simulink model "Quaternions_Method_merge"  (R2021b)
settings: Solver=VariableStepAuto  StartTime=0.0  StopTime=Time  FixedStep=1e-1  RelTol=1e-13  AbsTol=1e-8
values from neighbouring files (symbols this model uses):
  a = 8.6251e+06    (= 8625100)    [Main.m]
  c = 299792*10^3    (= 299792000)    [Main.m]
  e = 0.1195    [Main.m]
  f_mag = 5    [Main.m]
  H_0 = sqrt((g_1_0)^2 + (g_1_1)^2 + (h_1_1)^2)    [Main.m]
  i = 0.3815    [Main.m]
  MB = [2000; 0.3; 1; 0.12].*1e-2    [Main.m]
  mr = 1.2 * 0.0001    (= 0.00012)    [Main.m]
  muP = G*Mt    (= 398527110340000)    [Main.m]
  omega_0 = [om_x, om_y, om_z]    [Main.m]
  p_acc = deg2rad(5)    [Main.m]
  RD = 0.1*ones(1,10)    [Main.m]
  RS_MB = 0.5    [Main.m]
  RS_SP = 0.1    [Main.m]
  SP = [2000; 0.3; 1; 0.12].*1e-2    [Main.m]
  theta0 = 0    [Main.m]
  w_E = (2*pi)/(24*3600)    (= 7.27220521664e-05)    [Main.m]
undefined symbols (not defined in the file or in its folder): A_BN_0, A_rw, A_rw_star, magnitude, sig_b, sig_n, T, t_sample
libraries: matrix_library x14, vrlib x8, simulink x2, simulink_extras x1
(part 4 of 4)

== system Quaternions_Method_merge/Enviroment/Solar Radiation Perturbation/Sum forces/determine highlighted area/creazione della matrice che ha per colonne i vettori distanza tra il CM del MB e i centri geom delle aree illuminate dal sole /creazione raggi vettore tra CM MB e centro facce illuminate della faccia che ha come normale l'asse j/If Action Subsystem3 ==
  Areas_vect : Inport
  MB : Inport  Port=2
  Action Port : ActionPort  ActionPortLabel=if(u1<0 & u2<0)
  Add : Sum  Inputs=+|-
  Add1 : Sum  Inputs=+|-
  Add2 : Sum
  Demux : Demux  Outputs=3
  Demux2 : Demux
  Divide : Product  Inputs=*/
  Divide1 : Product  Inputs=*/
  Gain{,1..3} (4 alike) : Gain  Gain=1/2
  Gain4 : Gain  Gain=-1
  Gain5 : Gain  Gain=-1
  Ground : Ground
  Ground1 : Ground
  Mux : Mux  Inputs=3
  Mux1 : Mux  Inputs=3
  Reshape : Reshape  OutputDimensionality=Column vector (2-D)
  Reshape2 : Reshape  OutputDimensionality=Column vector (2-D)
  Reshape3 : Reshape  OutputDimensionality=Column vector (2-D)
  Terminator{1..2,8..9} (4 alike) : Terminator
  r_cface_cluce_x_neg_z_neg : Outport
  wires:
  Add1/1 -> Gain4/1
  Gain4/1 -> Mux1/1
  Demux/3 -> Terminator8/1
  Demux/1 -> Terminator9/1
  Add2/1 -> r_cface_cluce_x_neg_z_neg/1
  Reshape3/1 -> Add2/2
  Reshape2/1 -> Add2/1
  [a_MB] -> Gain2/1
  Divide1/1 -> Gain3/1
  Gain2/1 -> Add1/1
  Gain3/1 -> Add1/2
  Ground/1 -> Mux1/3, Mux1/2
  Mux1/1 -> Reshape3/1  "raggio vettore che collega il centro geom della faccia con il centro geom della faccia illuminata dal sole lungo -i"
  [h_MB] -> Divide1/2
  Reshape/1 -> Demux/1
  Ground1/1 -> Mux/1, Mux/2
  Areas_vect/1 -> Reshape/1
  [a_MB] -> Divide/2
  Gain/1 -> Add/1
  [h_MB] -> Gain/1
  Demux/2 -> Divide/1, Divide1/1
  Gain1/1 -> Add/2
  Mux/1 -> Reshape2/1  "raggio vettore che collega il centro geom della faccia con il centro geom della faccia illuminata dal sole lungo -k"
  Divide/1 -> Gain1/1
  Add/1 -> Gain5/1
  Gain5/1 -> Mux/3
  Demux2/1 -> Terminator2/1
  Demux2/2 -> [a_MB]
  MB/1 -> Demux2/1
  Demux2/3 -> Terminator1/1
  Demux2/4 -> [h_MB]

== system Quaternions_Method_merge/Enviroment/Solar Radiation Perturbation/Sum forces/determine highlighted area/creazione della matrice che ha per colonne i vettori distanza tra il CM del MB e i centri geom delle aree illuminate dal sole /creazione raggi vettore tra CM MB e centro facce illuminate della faccia che ha come normale l'asse j/If Action Subsystem4 ==
  Action Port : ActionPort  ActionPortLabel=else
  Constant : Constant  Value=[0;0;0]
  Out1 : Outport
  wires:
  Constant/1 -> Out1/1

== system Quaternions_Method_merge/Enviroment/Solar Radiation Perturbation/Sum forces/determine highlighted area/creazione della matrice che ha per colonne i vettori distanza tra il CM del MB e i centri geom delle aree illuminate dal sole /creazione raggi vettore tra CM MB e centro facce illuminate della faccia che ha come normale l'asse j/If Action Subsystem5 ==
  Action Port : ActionPort  ActionPortLabel=else
  Constant : Constant  Value=[0;0;0]
  Out1 : Outport
  wires:
  Constant/1 -> Out1/1

== system Quaternions_Method_merge/Enviroment/Solar Radiation Perturbation/Sum forces/determine highlighted area/creazione della matrice che ha per colonne i vettori distanza tra il CM del MB e i centri geom delle aree illuminate dal sole /creazione raggi vettore tra CM MB e centro facce illuminate della faccia che ha come normale l'asse j/If Action Subsystem6 ==
  Action Port : ActionPort  ActionPortLabel=else
  Constant : Constant  Value=[0;0;0]
  Out1 : Outport
  wires:
  Constant/1 -> Out1/1

== system Quaternions_Method_merge/Enviroment/Solar Radiation Perturbation/Sum forces/determine highlighted area/creazione della matrice che ha per colonne i vettori distanza tra il CM del MB e i centri geom delle aree illuminate dal sole /creazione raggi vettore tra CM MB e centro facce illuminate della faccia che ha come normale l'asse j/If Action Subsystem7 ==
  Action Port : ActionPort  ActionPortLabel=else
  Constant : Constant  Value=[0;0;0]
  Out1 : Outport
  wires:
  Constant/1 -> Out1/1

== system Quaternions_Method_merge/Enviroment/Solar Radiation Perturbation/Sum forces/determine highlighted area/creazione della matrice che ha per colonne i vettori distanza tra il CM del MB e i centri geom delle aree illuminate dal sole /creazione raggi vettore tra CM MB e centro facce illuminate della faccia che ha come normale l'asse j/creating distance between cm MB and centro geom lato1 ==
  MB : Inport
  Demux : Demux
  Ground : Ground
  Mux : Mux  Inputs=3
  Reshape : Reshape  OutputDimensionality=Column vector (2-D)
  Terminator : Terminator
  Terminator1 : Terminator
  Terminator2 : Terminator
  Out1 : Outport
  wires:
  Reshape/1 -> Out1/1
  Mux/1 -> Reshape/1
  Demux/4 -> Mux/3
  MB/1 -> Demux/1
  Demux/1 -> Terminator/1
  Demux/2 -> Terminator1/1
  Demux/3 -> Terminator2/1
  Ground/1 -> Mux/1, Mux/2

== system Quaternions_Method_merge/Enviroment/Solar Radiation Perturbation/Sum forces/determine highlighted area/creazione della matrice che ha per colonne i vettori distanza tra il CM del MB e i centri geom delle aree illuminate dal sole /creazione raggi vettore tra CM MB e centro facce illuminate della faccia che ha come normale l'asse k/If Action Subsystem ==
  Areas_vect : Inport
  MB : Inport  Port=2
  Action Port : ActionPort  ActionPortLabel=if(u1>0 & u2>0)
  Add : Sum  Inputs=+|-
  Add1 : Sum  Inputs=+|-
  Add2 : Sum
  Demux : Demux  Outputs=3
  Demux1 : Demux  Outputs=3
  Demux2 : Demux
  Divide : Product  Inputs=*/
  Divide1 : Product  Inputs=*/
  Gain{,1..3} (4 alike) : Gain  Gain=1/2
  Ground : Ground
  Ground1 : Ground
  Mux : Mux  Inputs=3
  Mux1 : Mux  Inputs=3
  Reshape{,1..3} (4 alike) : Reshape  OutputDimensionality=Column vector (2-D)
  Terminator{,1..3,8..9} (6 alike) : Terminator
  r_cface_cluce_xy_pos : Outport
  wires:
  Add/1 -> Mux/2
  Divide/1 -> Gain1/1
  Mux/1 -> Reshape2/1  "raggio vettore che collega il centro geom della faccia con il centro geom della faccia illuminata dal sole lungo j"
  Gain1/1 -> Add/2
  Demux/3 -> Divide/1
  [b_MB] -> Gain/1
  Gain/1 -> Add/1
  [a_MB] -> Divide/2
  Areas_vect/1 -> Reshape/1, Reshape1/1
  Ground1/1 -> Mux/1, Mux/3
  Reshape/1 -> Demux/1
  Add1/1 -> Mux1/1
  [b_MB] -> Divide1/2
  Mux1/1 -> Reshape3/1  "raggio vettore che collega il centro geom della faccia con il centro geom della faccia illuminata dal sole lungo x"
  Ground/1 -> Mux1/2, Mux1/3
  Demux1/3 -> Divide1/1
  Gain3/1 -> Add1/2
  Gain2/1 -> Add1/1
  Reshape1/1 -> Demux1/1
  Divide1/1 -> Gain3/1
  [a_MB] -> Gain2/1
  Reshape2/1 -> Add2/1
  Reshape3/1 -> Add2/2
  Add2/1 -> r_cface_cluce_xy_pos/1
  Demux1/1 -> Terminator/1
  Demux1/2 -> Terminator1/1
  Demux/1 -> Terminator9/1
  Demux/2 -> Terminator8/1
  MB/1 -> Demux2/1
  Demux2/1 -> Terminator2/1
  Demux2/2 -> [a_MB]
  Demux2/3 -> [b_MB]
  Demux2/4 -> Terminator3/1

== system Quaternions_Method_merge/Enviroment/Solar Radiation Perturbation/Sum forces/determine highlighted area/creazione della matrice che ha per colonne i vettori distanza tra il CM del MB e i centri geom delle aree illuminate dal sole /creazione raggi vettore tra CM MB e centro facce illuminate della faccia che ha come normale l'asse k/If Action Subsystem1 ==
  Areas_vect : Inport
  MB : Inport  Port=2
  Action Port : ActionPort  ActionPortLabel=if(u1>0 & u2<0)
  Add : Sum  Inputs=+|-
  Add1 : Sum  Inputs=+|-
  Add2 : Sum
  Demux : Demux  Outputs=3
  Demux1 : Demux  Outputs=3
  Demux2 : Demux
  Divide : Product  Inputs=*/
  Divide1 : Product  Inputs=*/
  Gain{,1..3} (4 alike) : Gain  Gain=1/2
  Gain4 : Gain  Gain=-1
  Ground : Ground
  Ground1 : Ground
  Mux : Mux  Inputs=3
  Mux1 : Mux  Inputs=3
  Reshape{,1..3} (4 alike) : Reshape  OutputDimensionality=Column vector (2-D)
  Terminator{,1..3,8..9} (6 alike) : Terminator
  r_cface_cluce_xpos_y_neg : Outport
  wires:
  Add/1 -> Gain4/1
  Divide/1 -> Gain1/1
  Mux/1 -> Reshape2/1  "raggio vettore che collega il centro geom della faccia con il centro geom della faccia illuminata dal sole lungo -j"
  Gain1/1 -> Add/2
  Demux/3 -> Divide/1
  Gain/1 -> Add/1
  Areas_vect/1 -> Reshape/1, Reshape1/1
  Ground1/1 -> Mux/1, Mux/3
  Reshape/1 -> Demux/1
  Mux1/1 -> Reshape3/1  "raggio vettore che collega il centro geom della faccia con il centro geom della faccia illuminata dal sole lungo i"
  Ground/1 -> Mux1/2, Mux1/3
  Demux1/3 -> Divide1/1
  Gain3/1 -> Add1/2
  Gain2/1 -> Add1/1
  Reshape1/1 -> Demux1/1
  Divide1/1 -> Gain3/1
  Reshape2/1 -> Add2/1
  Reshape3/1 -> Add2/2
  Add2/1 -> r_cface_cluce_xpos_y_neg/1
  Demux1/1 -> Terminator/1
  Demux1/2 -> Terminator1/1
  Demux/1 -> Terminator9/1
  Demux/2 -> Terminator8/1
  Gain4/1 -> Mux/2
  [a_MB] -> Divide/2
  [b_MB] -> Gain/1
  Add1/1 -> Mux1/1
  [b_MB] -> Divide1/2
  [a_MB] -> Gain2/1
  Demux2/1 -> Terminator2/1
  Demux2/2 -> [a_MB]
  MB/1 -> Demux2/1
  Demux2/3 -> [b_MB]
  Demux2/4 -> Terminator3/1

== system Quaternions_Method_merge/Enviroment/Solar Radiation Perturbation/Sum forces/determine highlighted area/creazione della matrice che ha per colonne i vettori distanza tra il CM del MB e i centri geom delle aree illuminate dal sole /creazione raggi vettore tra CM MB e centro facce illuminate della faccia che ha come normale l'asse k/If Action Subsystem2 ==
  Areas_vect : Inport
  MB1 : Inport  Port=2
  Action Port : ActionPort  ActionPortLabel=if(u1<0 & u2<0)
  Add : Sum  Inputs=+|-
  Add1 : Sum  Inputs=+|-
  Add2 : Sum
  Demux : Demux  Outputs=3
  Demux1 : Demux  Outputs=3
  Demux2 : Demux
  Divide : Product  Inputs=*/
  Divide1 : Product  Inputs=*/
  Gain{,1..3} (4 alike) : Gain  Gain=1/2
  Gain4 : Gain  Gain=-1
  Gain5 : Gain  Gain=-1
  Ground : Ground
  Ground1 : Ground
  Mux : Mux  Inputs=3
  Mux1 : Mux  Inputs=3
  Reshape{,1..3} (4 alike) : Reshape  OutputDimensionality=Column vector (2-D)
  Terminator{,1..3,8..9} (6 alike) : Terminator
  r_cface_cluce_xneg_y_neg : Outport
  wires:
  [a_MB] -> Divide1/2
  [b_MB] -> Gain2/1
  Add1/1 -> Gain5/1
  Gain4/1 -> Mux/1
  Add/1 -> Gain4/1
  [a_MB] -> Gain/1
  [b_MB] -> Divide/2
  Divide/1 -> Gain1/1
  Mux/1 -> Reshape2/1  "raggio vettore che collega il centro geom della faccia con il centro geom della faccia illuminata dal sole lungo -i"
  Gain1/1 -> Add/2
  Demux/3 -> Divide/1
  Gain/1 -> Add/1
  Areas_vect/1 -> Reshape/1, Reshape1/1
  Ground1/1 -> Mux/3, Mux/2
  Reshape/1 -> Demux/1
  Mux1/1 -> Reshape3/1  "raggio vettore che collega il centro geom della faccia con il centro geom della faccia illuminata dal sole lungo -j"
  Ground/1 -> Mux1/3, Mux1/1
  Demux1/3 -> Divide1/1
  Gain3/1 -> Add1/2
  Gain2/1 -> Add1/1
  Reshape1/1 -> Demux1/1
  Divide1/1 -> Gain3/1
  Reshape2/1 -> Add2/1
  Reshape3/1 -> Add2/2
  Add2/1 -> r_cface_cluce_xneg_y_neg/1
  Demux1/1 -> Terminator/1
  Demux1/2 -> Terminator1/1
  Demux/1 -> Terminator9/1
  Demux/2 -> Terminator8/1
  Gain5/1 -> Mux1/2
  Demux2/1 -> Terminator2/1
  Demux2/2 -> [a_MB]
  MB1/1 -> Demux2/1
  Demux2/3 -> [b_MB]
  Demux2/4 -> Terminator3/1

== system Quaternions_Method_merge/Enviroment/Solar Radiation Perturbation/Sum forces/determine highlighted area/creazione della matrice che ha per colonne i vettori distanza tra il CM del MB e i centri geom delle aree illuminate dal sole /creazione raggi vettore tra CM MB e centro facce illuminate della faccia che ha come normale l'asse k/If Action Subsystem3 ==
  Action Port : ActionPort  ActionPortLabel=else
  Constant : Constant  Value=[0;0;0]
  Out1 : Outport
  wires:
  Constant/1 -> Out1/1

== system Quaternions_Method_merge/Enviroment/Solar Radiation Perturbation/Sum forces/determine highlighted area/creazione della matrice che ha per colonne i vettori distanza tra il CM del MB e i centri geom delle aree illuminate dal sole /creazione raggi vettore tra CM MB e centro facce illuminate della faccia che ha come normale l'asse k/If Action Subsystem4 ==
  Areas_vect : Inport
  MB1 : Inport  Port=2
  Action Port : ActionPort  ActionPortLabel=if(u1<0 & u2>0)
  Add : Sum  Inputs=+|-
  Add1 : Sum  Inputs=+|-
  Add2 : Sum
  Demux : Demux  Outputs=3
  Demux1 : Demux  Outputs=3
  Demux2 : Demux
  Divide : Product  Inputs=*/
  Divide1 : Product  Inputs=*/
  Gain{,1..3} (4 alike) : Gain  Gain=1/2
  Gain4 : Gain  Gain=-1
  Ground : Ground
  Ground1 : Ground
  Mux : Mux  Inputs=3
  Mux1 : Mux  Inputs=3
  Reshape{,1..3} (4 alike) : Reshape  OutputDimensionality=Column vector (2-D)
  Terminator{,1..3,8..9} (6 alike) : Terminator
  r_cface_cluce_xneg_y_pos : Outport
  wires:
  Demux/2 -> Terminator8/1
  Demux/1 -> Terminator9/1
  Demux1/2 -> Terminator1/1
  Demux1/1 -> Terminator/1
  Add2/1 -> r_cface_cluce_xneg_y_pos/1
  Reshape3/1 -> Add2/2
  Reshape2/1 -> Add2/1
  Divide1/1 -> Gain3/1
  Reshape1/1 -> Demux1/1
  Gain2/1 -> Add1/1
  Gain3/1 -> Add1/2
  Demux1/3 -> Divide1/1
  Ground/1 -> Mux1/1, Mux1/3
  Mux1/1 -> Reshape3/1  "raggio vettore che collega il centro geom della faccia con il centro geom della faccia illuminata dal sole lungo j"
  Reshape/1 -> Demux/1
  Ground1/1 -> Mux/2, Mux/3
  Areas_vect/1 -> Reshape1/1, Reshape/1
  Gain/1 -> Add/1
  Demux/3 -> Divide/1
  Gain1/1 -> Add/2
  Mux/1 -> Reshape2/1  "raggio vettore che collega il centro geom della faccia con il centro geom della faccia illuminata dal sole lungo -i"
  Divide/1 -> Gain1/1
  [b_MB] -> Divide/2
  [a_MB] -> Gain/1
  Add/1 -> Gain4/1
  Gain4/1 -> Mux/1
  Add1/1 -> Mux1/2
  [b_MB] -> Gain2/1
  [a_MB] -> Divide1/2
  Demux2/1 -> Terminator2/1
  Demux2/2 -> [a_MB]
  MB1/1 -> Demux2/1
  Demux2/3 -> [b_MB]
  Demux2/4 -> Terminator3/1

== system Quaternions_Method_merge/Enviroment/Solar Radiation Perturbation/Sum forces/determine highlighted area/creazione della matrice che ha per colonne i vettori distanza tra il CM del MB e i centri geom delle aree illuminate dal sole /creazione raggi vettore tra CM MB e centro facce illuminate della faccia che ha come normale l'asse k/If Action Subsystem5 ==
  Action Port : ActionPort  ActionPortLabel=else
  Constant : Constant  Value=[0;0;0]
  Out1 : Outport
  wires:
  Constant/1 -> Out1/1

== system Quaternions_Method_merge/Enviroment/Solar Radiation Perturbation/Sum forces/determine highlighted area/creazione della matrice che ha per colonne i vettori distanza tra il CM del MB e i centri geom delle aree illuminate dal sole /creazione raggi vettore tra CM MB e centro facce illuminate della faccia che ha come normale l'asse k/If Action Subsystem6 ==
  Action Port : ActionPort  ActionPortLabel=else
  Constant : Constant  Value=[0;0;0]
  Out1 : Outport
  wires:
  Constant/1 -> Out1/1

== system Quaternions_Method_merge/Enviroment/Solar Radiation Perturbation/Sum forces/determine highlighted area/creazione della matrice che ha per colonne i vettori distanza tra il CM del MB e i centri geom delle aree illuminate dal sole /creazione raggi vettore tra CM MB e centro facce illuminate della faccia che ha come normale l'asse k/If Action Subsystem7 ==
  Action Port : ActionPort  ActionPortLabel=else
  Constant : Constant  Value=[0;0;0]
  Out1 : Outport
  wires:
  Constant/1 -> Out1/1

== system Quaternions_Method_merge/Enviroment/Solar Radiation Perturbation/Sum forces/determine highlighted area/creazione della matrice che ha per colonne i vettori distanza tra il CM del MB e i centri geom delle aree illuminate dal sole /creazione raggi vettore tra CM MB e centro facce illuminate della faccia che ha come normale l'asse k/creating distance between cm MB and centro geom lato1 ==
  MB : Inport
  Demux : Demux
  Ground : Ground
  Mux : Mux  Inputs=3
  Reshape : Reshape  OutputDimensionality=Column vector (2-D)
  Terminator : Terminator
  Terminator2 : Terminator
  Terminator3 : Terminator
  Out1 : Outport
  wires:
  Reshape/1 -> Out1/1
  Mux/1 -> Reshape/1
  MB/1 -> Demux/1
  Demux/1 -> Terminator/1
  Demux/2 -> Mux/1
  Demux/3 -> Terminator2/1
  Ground/1 -> Mux/2, Mux/3
  Demux/4 -> Terminator3/1

== matlab function Quaternions_Method_merge/Attitude determination/MATLAB Function ==
  data: K input; V output; D output
function [V, D] = fcn(K)
[V,D] = eig(K);
end
